simulink model "kp_contol_400"  (R2023a)
settings: Solver=VariableStepAuto  StartTime=0.0  StopTime=10.0  RelTol=1e-3
settings Model: Creator=TUBA  LastModifiedBy=TUBA

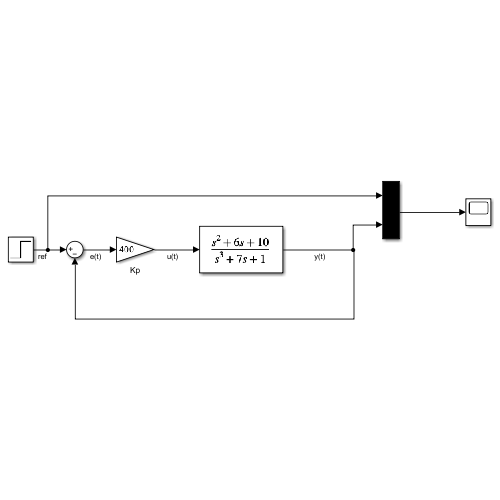
[thumbnail: Simulink's stored preview of the top-level diagram]
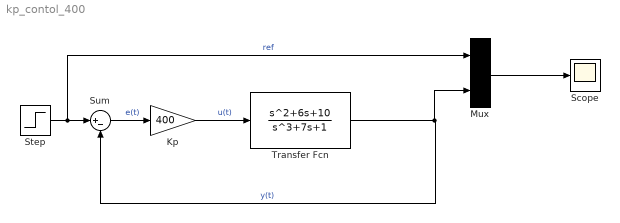
== system kp_contol_400 ==
  Kp : Gain  Gain=400
  Mux : Mux  Inputs=2
  Scope : Scope
  Step : Step  SampleTime=0
  Sum : Sum  Inputs=|+-
  Transfer Fcn : TransferFcn  Numerator=[1,6,10]  Denominator=[1,0,7,1]
  wires:
  Transfer Fcn/1 -> Mux/2, Sum/2  "y(t)"
  Kp/1 -> Transfer Fcn/1  "u(t)"
  Sum/1 -> Kp/1  "e(t)"
  Step/1 -> Mux/1, Sum/1  "ref"
  Mux/1 -> Scope/1
